simulink model "tetherInternalForces_th"  (R2018b)
settings: Solver=VariableStepAuto  StartTime=0.0  StopTime=0  RelTol=1e-3
values from neighbouring files (symbols this model uses):
  L = 90    [tetherInternalForces_ts.m]
  R1_o = [0 0 0]'    [tetherInternalForces_ts.m]
  Ri_o = zeros(3,N-2)    [tetherInternalForces_ts.m]
  Rn_o = [0 0 100]'    [tetherInternalForces_ts.m]
  V1_o = [0 0 0]'    [tetherInternalForces_ts.m]
  Vi_o = zeros(size(Ri_o))    [tetherInternalForces_ts.m]
  Vn_o = [0 0 0]'    [tetherInternalForces_ts.m]
libraries: tetherInternalForces_ul x1
settings Model: Creator=asiddiq2  LastModifiedBy=asiddiq2

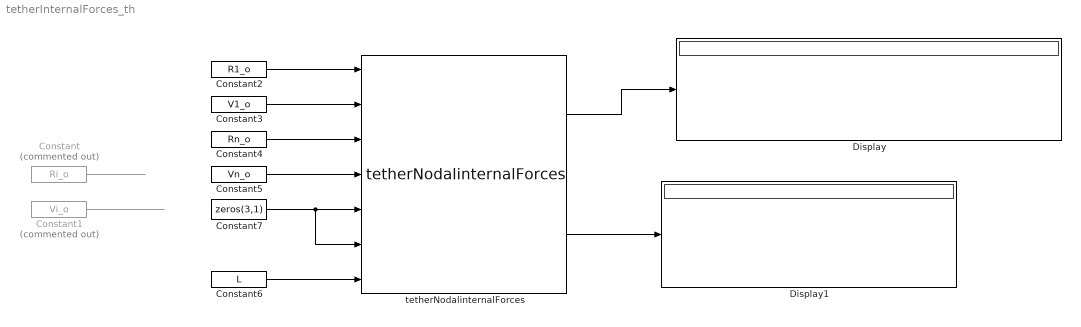
== system tetherInternalForces_th ==
  Constant : Constant  Commented=on  Value=Ri_o  VectorParams1D=off
  Constant1 : Constant  Commented=on  Value=Vi_o  VectorParams1D=off
  Constant2 : Constant  Value=R1_o  VectorParams1D=off
  Constant3 : Constant  Value=V1_o  VectorParams1D=off
  Constant4 : Constant  Value=Rn_o  VectorParams1D=off
  Constant5 : Constant  Value=Vn_o  VectorParams1D=off
  Constant6 : Constant  Value=L  VectorParams1D=off
  Constant7 : Constant  Value=zeros(3,1)  VectorParams1D=off
  Display : Display
  Display1 : Display
  tetherNodalinternalForces : tetherInternalForces_ul/tetherNodalinternalForces  massBdy=mass  numNode=N  diaTether=dia_t  youngsTether=E  zetaTether=zeta
  wires:
  Constant6/1 -> tetherNodalinternalForces/7
  tetherNodalinternalForces/1 -> Display/1
  Constant1/1 -> ?
  Constant/1 -> ?
  Constant2/1 -> tetherNodalinternalForces/1
  Constant3/1 -> tetherNodalinternalForces/2
  Constant5/1 -> tetherNodalinternalForces/4
  Constant4/1 -> tetherNodalinternalForces/3
  tetherNodalinternalForces/2 -> Display1/1
  Constant7/1 -> tetherNodalinternalForces/6, tetherNodalinternalForces/5
